simulink model "magballdemo"  (Simulink 7.6)
settings: Solver=ode45  StartTime=0.0  StopTime=10  RelTol=1e-3
PreLoadFcn:
  | magballdat
values from neighbouring files (symbols this model uses):
  beta = 0.001    [magballdat.m]
  L = 0.02    [magballdat.m]    (also in scd_aero_guid_dat.m = 0.0065; scdaircraftpad.m = LinearAircraft.values(:,:,17); scdsaturationDFpad.m = zpk([],[0 -1 -10],1))
  m = 0.1    [magballdat.m]
  R = 2    [magballdat.m]    (also in scd_aero_guid_dat.m = 287.26; scdboilerpad.m = diag([1e2,1e6]); scddcmotorpad.m = [2,1.8,2.2])
settings Model: Creator=The MathWorks Inc.  BufferReuse=off
settings DataIOCC: InitialState=x0  SignalLoggingName=logsOut
settings OptimizationCC: BlockReduction=off  InlineParams=on  InlineInvariantSignals=on  BufferReuse=off  InitFltsAndDblsToZero=on
settings DebuggingCC: SaveWithParameterizedLinksMsg=none  CheckExecutionContextPreStartOutputMsg=on  CheckExecutionContextRuntimeOutputMsg=on  SignalResolutionControl=TryResolveAllWithWarning  SolverPrmCheckMsg=none  MultiTaskDSMMsg=warning  StrictBusMsg=None
settings HardwareCC: TargetUnknown=on
settings GRTTargetCC: TargetFcnLib=ansi_tfl_tmw.mat

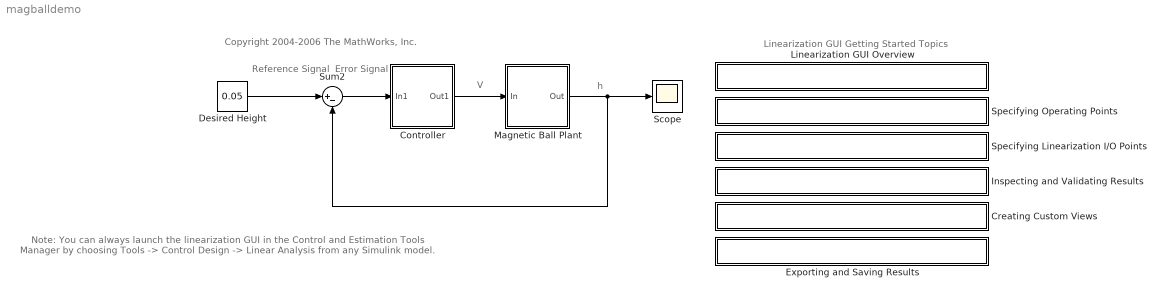
== system magballdemo ==
  note: Error
      | Signal
  note: Reference
      | Signal
  note: V
  note: h
  note: Linearization GUI Getting Started Topics
  note: Note: You can always launch the linearization GUI in the Control and Estimation Tools Manager
      | by choosing Tools -> Control Design -> Linear Analysis from any Simulink model.
  note: Copyright 2004-2006 The MathWorks, Inc.
  Controller : Subsystem
  Creating Custom Views : Subsystem  Priority=2
      settings: OpenFcn=scdguihelp('custom_views','HelpBrowser')
      mask Display: disp('Creating Custom Views')
  Desired Height : Constant  Value=0.05
  Exporting and Saving Results : Subsystem  Priority=2
      settings: OpenFcn=scdguihelp('exporting','HelpBrowser')
      mask Display: disp('Exporting and Saving Results')
  Inspecting and Validating Results : Subsystem  Priority=2
      settings: OpenFcn=scdguihelp('analyzing','HelpBrowser')
      mask Display: disp('Inspecting and Validating Results')
  Linearization GUI Overview : Subsystem  Priority=2
      settings: OpenFcn=scdguihelp('linearizing_models','HelpBrowser')
      mask Display: disp('Linearization GUI Overview')
  Magnetic Ball Plant : Subsystem
  Scope : Scope
  Specifying Linearization I/O Points : Subsystem  Priority=2
      settings: OpenFcn=scdguihelp('analysis_ios','HelpBrowser')
      mask Display: disp('Specifying Linearization I/O Points')
  Specifying Operating Points : Subsystem  Priority=2
      settings: OpenFcn=scdguihelp('op_points','HelpBrowser')
      mask Display: disp('Specifying Operating Points')
  Sum2 : Sum  Inputs=|+-
  wires:
  Magnetic Ball Plant/1(Out) -> Scope/1, Sum2/2
  Sum2/1 -> Controller/1(In1)
  Controller/1(Out1) -> Magnetic Ball Plant/1(In)
  Desired Height/1 -> Sum2/1

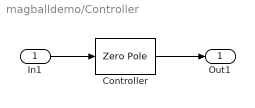
== system magballdemo/Controller ==
  In1 : Inport
  Controller : ZeroPole  Zeros=[-11.5000+5.7900i,-11.5000-5.7900i]  Poles=[0 -1000]  Gain=-3.3057e+004
  Out1 : Outport
  wires:
  In1/1 -> Controller/1
  Controller/1 -> Out1/1

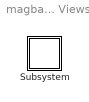
== system magballdemo/Creating Custom Views ==
  Subsystem : Subsystem

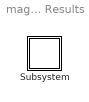
== system magballdemo/Exporting and Saving Results ==
  Subsystem : Subsystem

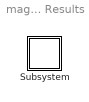
== system magballdemo/Inspecting and Validating Results ==
  Subsystem : Subsystem

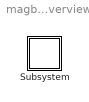
== system magballdemo/Linearization GUI Overview ==
  Subsystem : Subsystem

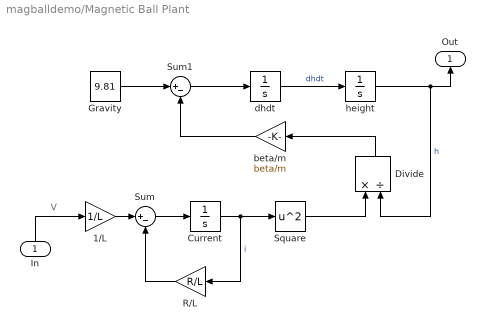
== system magballdemo/Magnetic Ball Plant ==
  note: V
  In : Inport
  1/L : Gain  Gain=1/L
  Current : Integrator  InitialCondition=7.0036
  Divide : Product  Inputs=*/
  Gravity : Constant  Value=9.81
  R/L : Gain  Gain=R/L
  Square : Math  Operator=square  SaturateOnIntegerOverflow=on
  Sum : Sum  Inputs=|+-
  Sum1 : Sum  Inputs=|+-
  beta/m : Gain  Gain=beta/m
  dhdt : Integrator
  height : Integrator  InitialCondition=0.05
  Out : Outport
  wires:
  dhdt/1 -> height/1  "dhdt"
  height/1 -> Out/1, Divide/2  "h"
  Sum/1 -> Current/1
  1/L/1 -> Sum/1
  R/L/1 -> Sum/2
  Current/1 -> Square/1, R/L/1  "i"
  Square/1 -> Divide/1
  Divide/1 -> beta/m/1
  Gravity/1 -> Sum1/1
  beta/m/1 -> Sum1/2
  Sum1/1 -> dhdt/1
  In/1 -> 1/L/1

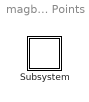
== system magballdemo/Specifying Linearization I/O Points ==
  Subsystem : Subsystem

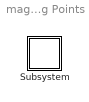
== system magballdemo/Specifying Operating Points ==
  Subsystem : Subsystem

== system magballdemo/Creating Custom Views/Subsystem ==

== system magballdemo/Exporting and Saving Results/Subsystem ==

== system magballdemo/Inspecting and Validating Results/Subsystem ==

== system magballdemo/Linearization GUI Overview/Subsystem ==

== system magballdemo/Specifying Linearization I/O Points/Subsystem ==

== system magballdemo/Specifying Operating Points/Subsystem ==
